simulink model "Quad_Sim_LQR_I"  (R2021b)
settings: Solver=ode4  StartTime=0.0  StopTime=Tfin  FixedStep=Ts  RelTol=1e-3
values from neighbouring files (symbols this model uses):
  CM = 8.881631641761697e-10    (= 8.88163164176e-10)    [run_simulation.m]
  Cr = 9.957365275903740e+03    (= 9957.3652759)    [run_simulation.m]
  CT = 5.724165806708346e-08    (= 5.72416580671e-08)    [run_simulation.m]
  f_sat = [22.7583, 3.4933e-05]    [run_simulation.m]
  g = 9.80665    [LQR_I_gain_tuning.m]    (also in run_simulation.m)
  Jxx = 0.010733986544371    (= 0.0107339865444)    [LQR_I_gain_tuning.m]    (also in run_simulation.m)
  Jyy = 0.011156873328260    (= 0.0111568733283)    [LQR_I_gain_tuning.m]    (also in run_simulation.m)
  Jzz = 0.022900774530029    (= 0.02290077453)    [LQR_I_gain_tuning.m]    (also in run_simulation.m)
  KPhi = [0.6433; 0.3714]    [run_simulation.m]
  KPsi = [0.1746; 0.1500; 0.0984]    [run_simulation.m]
  KTheta = [0.6455; 0.3734]    [run_simulation.m]
  Kxx = K(1,1:3)    [LQR_I_gain_tuning.m]    (also in run_simulation.m = [-0.4638; -0.5333; -0.1560])
  Kyy = K(2,4:6)    [LQR_I_gain_tuning.m]    (also in run_simulation.m = [0.4638; 0.5333; 0.1560])
  Kzz = K(3,7:9)    [LQR_I_gain_tuning.m]    (also in run_simulation.m = [-10.2854; -6.5162; -1.4903])
  m = 1.062    [LQR_I_gain_tuning.m]    (also in run_simulation.m)
  omega_b = 12.351763347436565    (= 12.3517633474)    [run_simulation.m]
  phi_sat = [0.8, -0.8]    [run_simulation.m]
  prop_dist = 0.170    (= 0.17)    [run_simulation.m]
  tauI = 0.5    [run_simulation.m]
  taux_sat = [1.3679, -1.3679]    [run_simulation.m]
  tauy_sat = [1.3679, -1.3679]    [run_simulation.m]
  tauz_sat = [0.35, -0.35]    [run_simulation.m]
  Th_init_vec = Th_init*ones(4,1)    [run_simulation.m]
  theta_sat = [0.8, -0.8]    [run_simulation.m]
  Tm = 0.245217435487778    (= 0.245217435488)    [run_simulation.m]
  Ts = 0.0001    [run_simulation.m]
  Ts_ct = 0.005    [LQR_I_gain_tuning.m]    (also in run_simulation.m)
  x0 = zeros(12,1)    [run_simulation.m]
settings Model: Creator=Juan Augusto Paredes  LastModifiedBy=Juan Augusto Paredes
settings SolverCC: AlgebraicLoopSolver=TrustRegion
settings DataIOCC: ReturnWorkspaceOutputs=off
settings DebuggingCC: SFMachineParentedDataDiag=warning  ArithmeticOperatorsInVariantConditions=warning
settings SFSimCC: SimUseLocalCustomCode=off  CustomCodeUndefinedFunction=UseInterfaceOnly
settings RTWCC: RTWUseLocalCustomCode=off

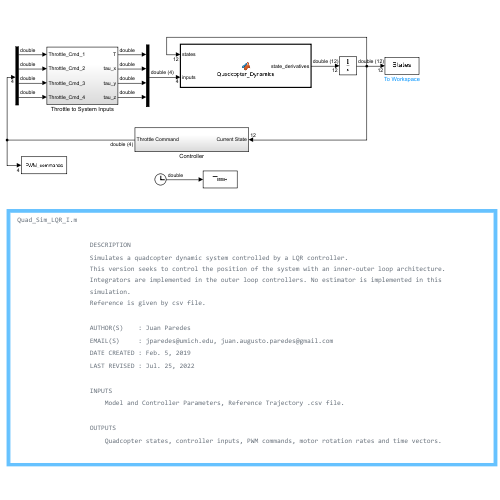
[thumbnail: Simulink's stored preview of the top-level diagram]
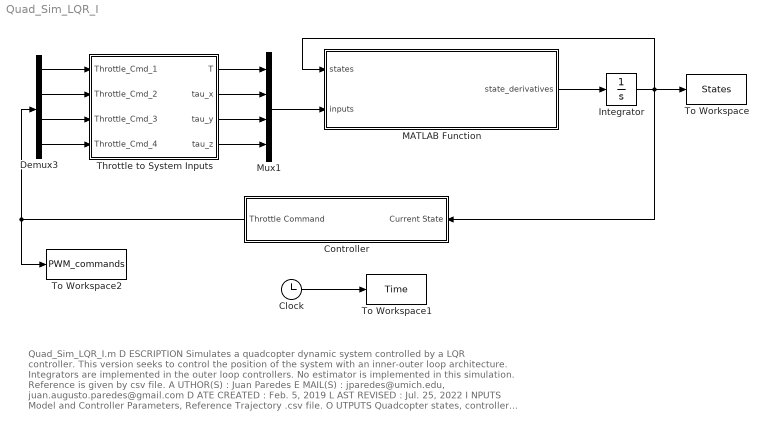
== system Quad_Sim_LQR_I ==
  note: Quad_Sim_LQR_I.m
      |
      | D ESCRIPTION
      |
      | Simulates a quadcopter dynamic system controlled by a LQR controller.
      | This version seeks to control the position of the system with an inner-outer loop architecture.
      | Integrators are implemented in the outer loop controllers. No estimator is implemented in this simulation.
      | Reference is given by csv file.
      |
      | A UTHOR(S) : Juan Paredes
      |
      | E MAIL(S) : jparedes@umich.edu, juan.augusto.paredes@gmail.com
      |
      | D ATE CREATED : Feb. 5, 2019
      |
      | L AST REVISED : Jul. 25, 2022
      |
      | I NPUTS
      |
      | Model and Controller Parameters, Reference Trajectory .csv file.
      |
      | O UTPUTS
      |
      | Quadcopter states, controller inputs, PWM commands, motor rotation rates and time vectors.
  Clock : Clock
  Controller : Subsystem
  Demux3 : Demux
  Integrator : Integrator  InitialCondition=x0
  MATLAB Function : MATLAB Function  TreatAsAtomicUnit=on
  Mux1 : Mux
  Throttle to System Inputs : Subsystem
  To Workspace : ToWorkspace  VariableName=States  SampleTime=-1
      settings: Save2DSignal=2-D array (concatenate along first dimension)
  To Workspace1 : ToWorkspace  VariableName=Time  SampleTime=-1
  To Workspace2 : ToWorkspace  VariableName=PWM_commands  SampleTime=-1
      settings: Save2DSignal=2-D array (concatenate along first dimension)
  wires:
  Throttle to System Inputs/1(T) -> Mux1/1
  Throttle to System Inputs/2(tau_x) -> Mux1/2
  Throttle to System Inputs/3(tau_y) -> Mux1/3
  Throttle to System Inputs/4(tau_z) -> Mux1/4
  Mux1/1 -> MATLAB Function/2(inputs)
  MATLAB Function/1(state_derivatives) -> Integrator/1
  Integrator/1 -> To Workspace/1, Controller/1(Current State), MATLAB Function/1(states)
  Controller/1(Throttle Command) -> To Workspace2/1, Demux3/1
  Demux3/1 -> Throttle to System Inputs/1(Throttle_Cmd_1)
  Demux3/2 -> Throttle to System Inputs/2(Throttle_Cmd_2)
  Demux3/3 -> Throttle to System Inputs/3(Throttle_Cmd_3)
  Demux3/4 -> Throttle to System Inputs/4(Throttle_Cmd_4)
  Clock/1 -> To Workspace1/1

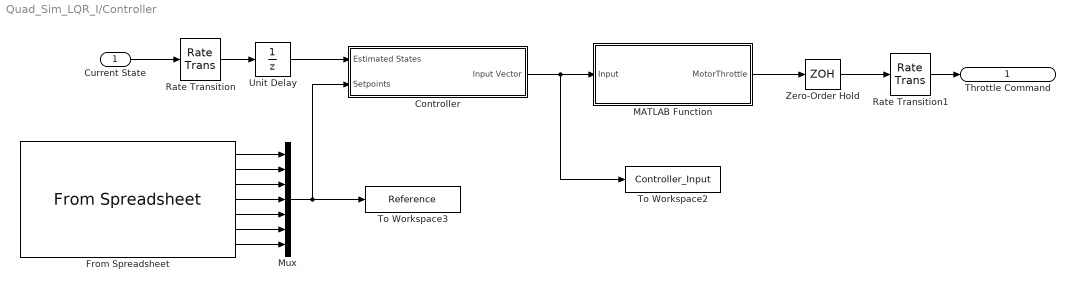
== system Quad_Sim_LQR_I/Controller ==
  Current State : Inport
  Controller : Subsystem
  From Spreadsheet : FromSpreadsheet  FileName=refTraj.csv  SheetName=refTraj  OutDataTypeStr=double  TreatFirstColumnAs=Data  SampleTime=Ts_ct  ExtrapolationBeforeFirstDataPoint=Hold first value  InterpolationWithinTimeRange=Zero order hold  ExtrapolationAfterLastDataPoint=Hold last value  OutputAfterLastPoint=Hold final value
  MATLAB Function : MATLAB Function  TreatAsAtomicUnit=on
  Mux : Mux  Inputs=7
  Rate Transition : RateTransition  InitialCondition=x0
  Rate Transition1 : RateTransition  InitialCondition=Th_init_vec
  To Workspace2 : ToWorkspace  VariableName=Controller_Input  SampleTime=Ts
      settings: Save2DSignal=2-D array (concatenate along first dimension)
  To Workspace3 : ToWorkspace  VariableName=Reference  SampleTime=Ts
      settings: Save2DSignal=2-D array (concatenate along first dimension)
  Unit Delay : UnitDelay  InitialCondition=x0  SampleTime=Ts_ct  HasFrameUpgradeWarning=on
  Zero-Order Hold : ZeroOrderHold  SampleTime=Ts_ct
  Throttle Command : Outport  VectorParamsAs1DForOutWhenUnconnected=off
  wires:
  Controller/1(Input Vector) -> MATLAB Function/1(Input), To Workspace2/1
  Current State/1 -> Rate Transition/1
  Unit Delay/1 -> Controller/1(Estimated States)
  From Spreadsheet/1 -> Mux/1
  From Spreadsheet/2 -> Mux/2
  From Spreadsheet/3 -> Mux/3
  From Spreadsheet/4 -> Mux/4
  From Spreadsheet/5 -> Mux/5
  From Spreadsheet/6 -> Mux/6
  From Spreadsheet/7 -> Mux/7
  Mux/1 -> To Workspace3/1, Controller/2(Setpoints)
  Rate Transition/1 -> Unit Delay/1
  Rate Transition1/1 -> Throttle Command/1
  MATLAB Function/1(MotorThrottle) -> Zero-Order Hold/1
  Zero-Order Hold/1 -> Rate Transition1/1

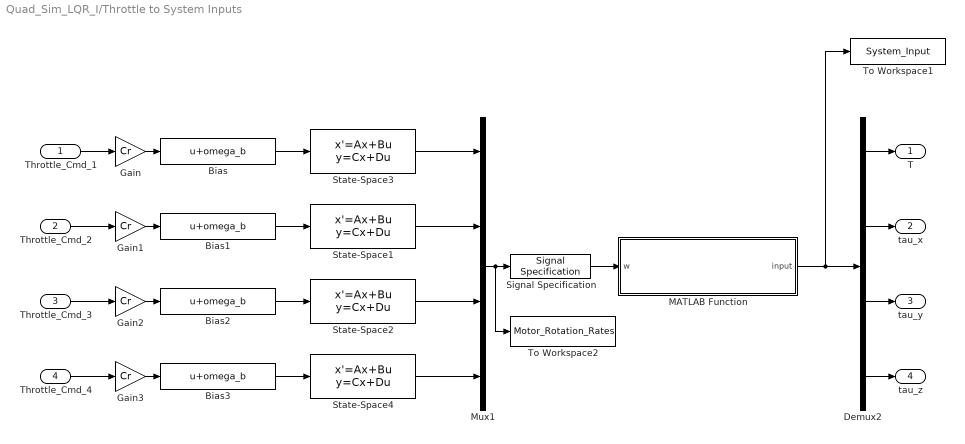
== system Quad_Sim_LQR_I/Throttle to System Inputs ==
  Throttle_Cmd_1 : Inport
  Throttle_Cmd_2 : Inport  Port=2
  Throttle_Cmd_3 : Inport  Port=3
  Throttle_Cmd_4 : Inport  Port=4
  Bias{,1..3} (4 alike) : Bias  Bias=omega_b
  Demux2 : Demux
  Gain{,1..3} (4 alike) : Gain  Gain=Cr
  MATLAB Function : MATLAB Function  TreatAsAtomicUnit=on
  Mux1 : Mux
  Signal Specification : SignalSpecification  Dimensions=[4, 1]
  State-Space{1..4} (4 alike) : StateSpace  A=-1/Tm  C=1/Tm  D=0  InitialCondition=Tm*sqrt(m*g/(4*CT))
  To Workspace1 : ToWorkspace  VariableName=System_Input  SampleTime=-1
      settings: Save2DSignal=2-D array (concatenate along first dimension)
  To Workspace2 : ToWorkspace  VariableName=Motor_Rotation_Rates  SampleTime=-1
      settings: Save2DSignal=2-D array (concatenate along first dimension)
  T : Outport  VectorParamsAs1DForOutWhenUnconnected=off
  tau_x : Outport  Port=2  VectorParamsAs1DForOutWhenUnconnected=off
  tau_y : Outport  Port=3  VectorParamsAs1DForOutWhenUnconnected=off
  tau_z : Outport  Port=4  VectorParamsAs1DForOutWhenUnconnected=off
  wires:
  Throttle_Cmd_1/1 -> Gain/1
  Gain/1 -> Bias/1
  Gain1/1 -> Bias1/1
  Throttle_Cmd_2/1 -> Gain1/1
  Gain2/1 -> Bias2/1
  Throttle_Cmd_3/1 -> Gain2/1
  Gain3/1 -> Bias3/1
  Throttle_Cmd_4/1 -> Gain3/1
  Bias/1 -> State-Space3/1
  Bias1/1 -> State-Space1/1
  Bias2/1 -> State-Space2/1
  Bias3/1 -> State-Space4/1
  State-Space3/1 -> Mux1/1
  State-Space1/1 -> Mux1/2
  State-Space2/1 -> Mux1/3
  State-Space4/1 -> Mux1/4
  Signal Specification/1 -> MATLAB Function/1(w)
  Mux1/1 -> To Workspace2/1, Signal Specification/1
  MATLAB Function/1(input) -> To Workspace1/1, Demux2/1
  Demux2/1 -> T/1
  Demux2/2 -> tau_x/1
  Demux2/3 -> tau_y/1
  Demux2/4 -> tau_z/1

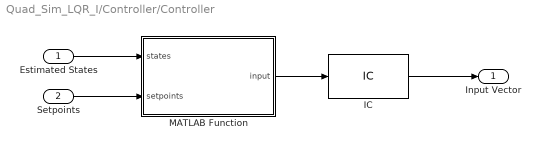
== system Quad_Sim_LQR_I/Controller/Controller ==
  Estimated States : Inport
  Setpoints : Inport  Port=2
  IC : InitialCondition  Value=[0;0;m*g; 0; 0; 0]
  MATLAB Function : MATLAB Function  TreatAsAtomicUnit=on
  Input Vector : Outport  VectorParamsAs1DForOutWhenUnconnected=off
  wires:
  Estimated States/1 -> MATLAB Function/1(states)
  MATLAB Function/1(input) -> IC/1
  IC/1 -> Input Vector/1
  Setpoints/1 -> MATLAB Function/2(setpoints)

== matlab function Quad_Sim_LQR_I/Throttle to System Inputs/MATLAB Function ==
  data: w input; input output; prop_dist parameter; CT parameter; CM parameter
function input = rotationalRateToControlInputs(w, prop_dist, CT, CM)

sq_d_CT = (sqrt(2)/2)*prop_dist*CT;

input = [CT, CT, CT, CT;...
    -sq_d_CT, -sq_d_CT, sq_d_CT, sq_d_CT;...
    sq_d_CT, -sq_d_CT, -sq_d_CT, sq_d_CT;...
    CM, -CM, CM, -CM]*(w.^2);

== matlab function Quad_Sim_LQR_I/MATLAB Function ==
  data: states input size=12; inputs input size=4; state_derivatives output size=12; m parameter size=1; Jxx parameter size=1; Jyy parameter size=1; Jzz parameter size=1; g parameter size=1
function state_derivatives = Quadcopter_Dynamics(states, inputs, m, Jxx, Jyy, Jzz, g)

%States: X, Y, Z, Xdot, Ydot, Zdot, phi, theta, psi, Body Pitch Rate, Body Roll Rate, Body Yaw Rate

%Inputs: Total thrust T, 3D Torque (tauX, tauY, tauZ)

%3D position with respect to inertial coordinate frame
x = states(1);
y = states(2);
z = states(3);

%3D velocities with respect to inertial coordinate frame
xdot = states(4);
ydot = states(5);
zdot = states(6);

%Euler angles with respect to inertial coordinate frame
phi = states(7);
theta = states(8);
psi = states(9);

%Rotation rate with respect to body frame
omega_xb = states(10);
omega_yb = states(11);
omega_zb = states(12);

T = inputs(1);      %Total thrust
tauX = inputs(2);   %Torque around X axis
tauY = inputs(3);   %Torque around Y axis
tauZ = inputs(4);   %Torque around Z axis

state_derivatives = zeros(12,1);

%3D velocities with respect to inertial coordinate frame
state_derivatives(1) = xdot;
state_derivatives(2) = ydot;
state_derivatives(3) = zdot;

%3D accelerations with respect to inertial coordinate frame

state_derivatives(4) = -(T/m)*(cos(psi)*sin(theta)*cos(phi) + sin(psi)*sin(phi));
state_derivatives(5) = -(T/m)*(sin(psi)*sin(theta)*cos(phi) - cos(psi)*sin(phi));
state_derivatives(6) = g - (T/m)*(cos(theta)*cos(phi)); 

%Euler angles velocities with respect to inertial coordinate frame

state_derivatives(7) = omega_xb + omega_yb*tan(theta)*sin(phi) + omega_zb*tan(theta)*cos(phi);
state_derivatives(8) = omega_yb*cos(phi) - omega_zb*sin(phi);
state_derivatives(9) = omega_yb*(sin(phi)/cos(theta)) + omega_zb*(cos(phi)/cos(theta));

%Rotation acceleration with respect to body frame
state_derivatives(10) = tauX/Jxx + ((Jyy-Jzz)/Jxx)*omega_yb*omega_zb;
state_derivatives(11) = tauY/Jyy + ((Jzz-Jxx)/Jyy)*omega_xb*omega_zb;
state_derivatives(12) = tauZ/Jzz + ((Jxx-Jyy)/Jzz)*omega_xb*omega_yb;

== matlab function Quad_Sim_LQR_I/Controller/MATLAB Function ==
  settings: updateMethod=DISCRETE  sampleTime=Ts_ct
  data: Input input size=6; MotorThrottle output size=4; prop_dist parameter; CT parameter; CM parameter; Cr parameter; omega_b parameter
function MotorThrottle = InputToMotorThrottle(Input, prop_dist, CT, CM, Cr, omega_b)

sq_d_CT = sqrt(2)/(4*prop_dist*CT);
CT_var = 1/(4*CT);
CM_var = 1/(4*CM);

Input_u = Input(3:6);

omega_des_sq = [CT_var -sq_d_CT sq_d_CT CM_var;...
    CT_var -sq_d_CT -sq_d_CT -CM_var;...
    CT_var sq_d_CT -sq_d_CT CM_var;...
    CT_var sq_d_CT sq_d_CT -CM_var]*Input_u;

omega_des_sq = min(max(omega_des_sq, omega_b^2),(Cr + omega_b)^2);

omega_des = sqrt(omega_des_sq);

MotorThrottle = min(max((omega_des - omega_b)/Cr,0),1);

== matlab function Quad_Sim_LQR_I/Controller/Controller/MATLAB Function ==
  settings: updateMethod=DISCRETE  sampleTime=Ts_ct
  data: states input size=12; setpoints input size=7; input output size=6; Kxx parameter; Kyy parameter; Kzz parameter; KPsi parameter; KPhi parameter; KTheta parameter; m parameter; g parameter; tauI parameter; theta_sat parameter; phi_sat parameter; f_sat parameter; taux_sat parameter; tauy_sat parameter; tauz_sat parameter; Ts_ct parameter
function input = LQRController(states, setpoints, Kxx, Kyy, Kzz, KPsi, KPhi, KTheta, m, g, tauI, theta_sat, phi_sat, f_sat, taux_sat, tauy_sat, tauz_sat, Ts_ct)

persistent xI
persistent yI
persistent zI
persistent psiI

persistent x_prev
persistent y_prev
persistent z_prev
persistent psi_prev

persistent x_int_res
persistent y_int_res
persistent z_int_res
persistent psi_int_res

if isempty(xI)
   
   xI = 0;
   yI = 0;
   zI = 0;
   psiI = 0;
   
   x_prev = [0;0];
   y_prev = [0;0];
   z_prev = [0;0];
   psi_prev = [0;0];
   
   x_int_res = 0;
   y_int_res = 0;
   z_int_res = 0;
   psi_int_res = 0;
   
end

%3D position with respect to inertial coordinate frame
x = states(1);
y = states(2);
z = states(3);

%3D velocities with respect to inertial coordinate frame
xdot = states(4);
ydot = states(5);
zdot = states(6);

%Euler angles with respect to inertial coordinate frame
phi = states(7);
theta = states(8);
psi = states(9);

%Rotation rate with respect to body frame

omega_xb = states(10);
omega_yb = states(11);
omega_zb = states(12);

X_des = setpoints(1);
Y_des = setpoints(2);
Z_des = setpoints(3);
Xdot_des = setpoints(4);
Ydot_des = setpoints(5);
Zdot_des = setpoints(6);
Psi_des = setpoints(7);

X_des_rel = cos(psi)*X_des + sin(psi)*Y_des;
Y_des_rel = -sin(psi)*X_des + cos(psi)*Y_des;
Xdot_des_rel = cos(psi)*Xdot_des + sin(psi)*Ydot_des;
Ydot_des_rel = -sin(psi)*Xdot_des + cos(psi)*Ydot_des;
X_rel = cos(psi)*x + sin(psi)*y;
Y_rel = -sin(psi)*x + cos(psi)*y;
Xdot_rel = cos(psi)*xdot + sin(psi)*ydot;
Ydot_rel = -sin(psi)*xdot + cos(psi)*ydot;

z_des_act = Z_des;
psi_des_act = Psi_des;

[Theta_des, xI, x_prev, x_int_res] = IntAntiWindup([X_des_rel - X_rel; Xdot_des_rel-Xdot_rel], Kxx, tauI, theta_sat(2), theta_sat(1), xI, x_prev, x_int_res, Ts_ct);

[Phi_des, yI, y_prev, y_int_res] = IntAntiWindup([Y_des_rel - Y_rel; Ydot_des_rel-Ydot_rel], Kyy, tauI, phi_sat(2), phi_sat(1), yI, y_prev, y_int_res, Ts_ct);

f_bias = m*g/(max((cos(theta)*cos(phi)),0.01));
[f, zI, z_prev, z_int_res] = IntAntiWindup([z_des_act - z; Zdot_des - zdot], Kzz, tauI, f_sat(2) - f_bias, f_sat(1) - f_bias, zI, z_prev, z_int_res, Ts_ct);
f = f + f_bias;

tauY = KTheta'*[Theta_des - theta; -omega_yb];
tauY = max(min(tauY, tauy_sat(1)), tauy_sat(2));

tauX = KPhi'*[Phi_des - phi; -omega_xb];
tauX = max(min(tauX, taux_sat(1)), taux_sat(2));

[tauZ, psiI, psi_prev, psi_int_res] = IntAntiWindup([psi_des_act - psi; -omega_zb], KPsi, tauI, tauz_sat(2), tauz_sat(1), psiI, psi_prev, psi_int_res, Ts_ct);

input = [Phi_des; Theta_des; f; tauX; tauY; tauZ];

end

function [u, state_int, state_prev, int_res] = IntAntiWindup(state, K, tau, minU, maxU, state_int_0, state_prev_0, int_res_0, Ts)
    
    error = state(1);
    states_dot = (state - state_prev_0)/Ts;
    aug_state = [states_dot;error];
    feedback = K'*aug_state;
    
    int_var = feedback + int_res_0;
    state_int = state_int_0 + Ts*(int_var);
    u = max(min(state_int, maxU), minU);
    int_res = tau*(u - state_int);
    state_prev = state;
    
end
